simulink model "task3"  (R2023b)
settings: Solver=FixedStepDiscrete  StartTime=0.0  StopTime=120  FixedStep=5e-5  RelTol=1e-3
PreLoadFcn:
  | Simulink.defineIntEnumType('windowCommand', {'Off','Speed1','Speed2','Speed3'},[0,1,2,3])
undefined symbols (not defined in the file or in its folder): designMultirateFIR
libraries: dspmlti4 x1, dspfdesign x1, slpidlib x1
settings Model: Creator=kz1nz0  LastModifiedBy=helme

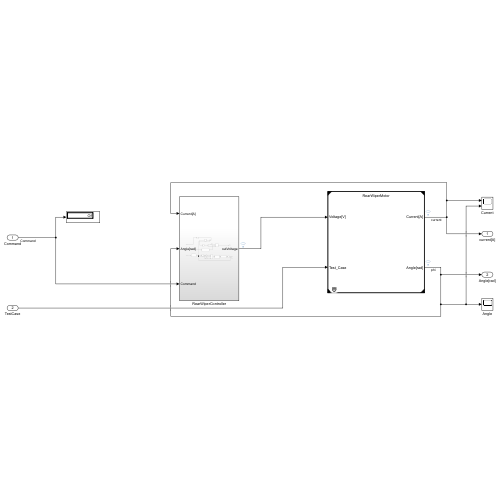
[thumbnail: Simulink's stored preview of the top-level diagram]
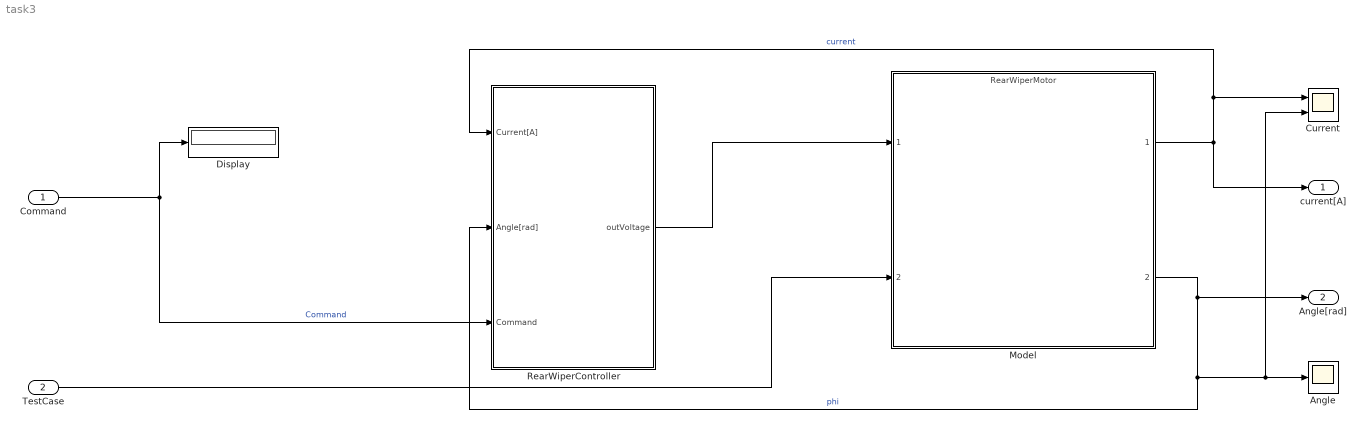
== system task3 ==
  Command : Inport  OutDataTypeStr=Enum: windowCommand
  TestCase : Inport  Port=2  OutDataTypeStr=int8
  Angle : Scope
  Current : Scope  NumInputPorts=2
  Display : Display
  Model : ModelReference  ModelNameDialog=RearWiperMotor.slxp  ModelReferenceVersion=19.15  CopyOfModelProtected=on
  RearWiperController : Subsystem
  current[A] : Outport
  Angle[rad] : Outport  Port=2
  wires:
  TestCase/1 -> Model/2
  Model/1 -> RearWiperController/1(Current[A]), Current/1, current[A]/1  "current"
  Model/2 -> Current/2, Angle/1, RearWiperController/2(Angle[rad]), Angle[rad]/1  "phi"
  RearWiperController/1(outVoltage) -> Model/1
  Command/1 -> Display/1, RearWiperController/3(Command)  "Command"

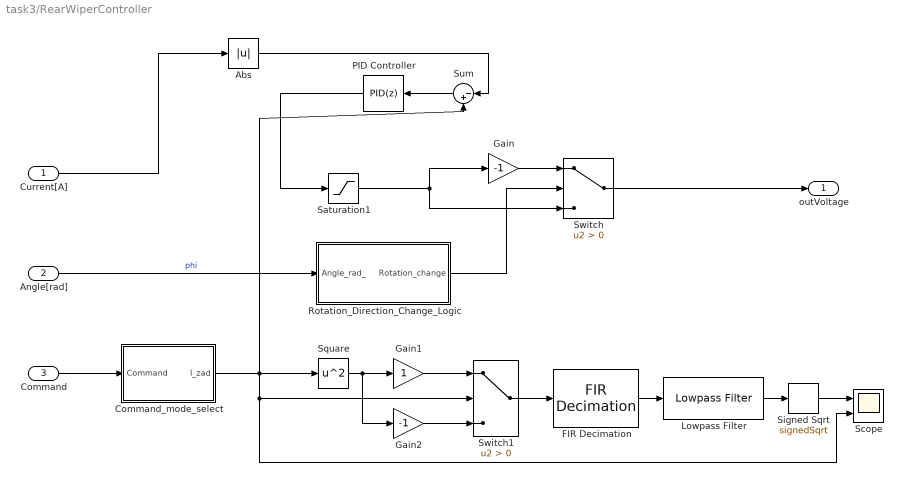
== system task3/RearWiperController ==
  Current[A] : Inport
  Angle[rad] : Inport  Port=2
  Command : Inport  Port=3  OutDataTypeStr=Enum: windowCommand
  Abs : Abs  SaturateOnIntegerOverflow=off
  Command_mode_select : Stateflow chart  TreatAsAtomicUnit=on
  FIR Decimation : dspmlti4/FIR Decimation  FilterSource=Auto  h=designMultirateFIR(1,2)  D=15  filtStruct=Direct form  FilterObject=FDECIM  framing=Enforce single-rate processing  AllowArbitraryInputLength=off  inputOffset=0  outputBufInitCond=0  roundingMode=Floor  overflowMode=off  firstCoeffDataTypeStr=Inherit: Same word length as input  firstCoeffMin=[]  firstCoeffMax=[]  firstCoeffLastDataTypeStr=Inherit: Same word length as input  outputDataTypeStr=Inherit: Same as accumulator  outputMin=[]  outputMax=[]  outputLastDataTypeStr=Inherit: Same as accumulator
  Gain : Gain  Gain=-1
  Gain1 : Gain
  Gain2 : Gain  Gain=-1
  Lowpass Filter : dspfdesign/Lowpass Filter  FilterType=FIR  DesignForMinimumOrder=on  FilterOrder=50  PassbandFrequency=8e3  StopbandFrequency=12e3  PassbandRipple=0.1  StopbandAttenuation=80  SampleRateMode=Specify on dialog  SampleRate=44100  SimulateUsing=Interpreted execution  roundingMode=Floor  coeffsDataTypeStr=fixdt(1,16)
  PID Controller : slpidlib/PID Controller  Controller=PID  Form=Parallel  TimeDomain=Discrete-time  UseExternalTs=off  SampleTime=-1  IntegratorMethod=Forward Euler  FilterMethod=Forward Euler  ControllerParametersSource=internal  P=20  I=0  UseKiTs=off  D=2  N=100  UseFilter=on  TunerSelectOption=Transfer Function Based (PID Tuner App)  InitialConditionSource=internal  InitialConditionForIntegrator=0  InitialConditionForFilter=0  DifferentiatorICPrevScaledInput=0  ExternalReset=none  TrackingMode=off  Kt=1  LimitOutput=off  SatLimitsSource=internal  UpperSaturationLimit=inf  LowerSaturationLimit=-inf  LinearizeAsGain=on  AntiWindupMode=none  Kb=1  LimitIntegrator=off  UpperIntegratorSaturationLimit=inf  LowerIntegratorSaturationLimit=-inf  POutMin=[]  POutMax=[]  IOutMin=[]  IOutMax=[]  DOutMin=[]  DOutMax=[]  NOutMin=[]  NOutMax=[]  SumOutMin=[]  SumOutMax=[]  SaturationOutMin=[]  SaturationOutMax=[]  PParamMin=[]  PParamMax=[]  IParamMin=[]  IParamMax=[]  DParamMin=[]  DParamMax=[]  NParamMin=[]  NParamMax=[]  KbParamMin=[]  KbParamMax=[]  KtParamMin=[]  KtParamMax=[]  KbOutMin=[]  KbOutMax=[]  KtOutMin=[]  KtOutMax=[]  IntegratorOutMin=[]  IntegratorOutMax=[]  FilterOutMin=[]  FilterOutMax=[]  SumI1OutMin=[]  SumI1OutMax=[]  SumI2OutMin=[]  SumI2OutMax=[]  SumI3OutMin=[]  SumI3OutMax=[]  SumI4OutMin=[]  SumI4OutMax=[]  SumDOutMin=[]  SumDOutMax=[]  DifferentiatorOutMin=[]  DifferentiatorOutMax=[]  FilterDiffOutCoefMin=[]  FilterDiffOutCoefMax=[]  ReciprocalOutMin=[]  ReciprocalOutMax=[]  SumDenOutMin=[]  SumDenOutMax=[]  SumNumOutMin=[]  SumNumOutMax=[]  DivideOutMin=[]  DivideOutMax=[]  UdiffTsProdOutMin=[]  UdiffTsProdOutMax=[]  NTsProdOutMin=[]  NTsProdOutMax=[]  UintegralTsProdOutMin=[]  UintegralTsProdOutMax=[]  UngainTsProdOutMin=[]  UngainTsProdOutMax=[]  ClampingZeroOutDataTypeStr=Inherit: Inherit via back propagation  ClampingZeroOutMin=[]  ClampingZeroOutMax=[]  FilterDenConstantOutDataTypeStr=Inherit: Inherit via back propagation  FilterDenConstantOutMin=[]  FilterDenConstantOutMax=[]  PCopyOutDataTypeStr=Inherit: Inherit via back propagation  PCopyOutMin=[]  PCopyOutMax=[]  NCopyOutDataTypeStr=Inherit: Inherit via back propagation  NCopyOutMin=[]  NCopyOutMax=[]  IntegratorContinuousStateAttributes=''  IntegratorStateMustResolveToSignalObject=off  IntegratorRTWStateStorageClass=Auto  FilterContinuousStateAttributes=''  FilterStateMustResolveToSignalObject=off  FilterRTWStateStorageClass=Auto  ParallelPVariant=InternalParameters  IdealPVariant=Disabled  IVariant=InternalParameters  DVariant=InternalParameters  IntegratorVariant=Discrete  SatVariant=Disabled  AWVariant=Passthrough  PCopyVariant=Disabled  TRVariant=Disabled  FdbkBlocksVariant=Forward  IdealPFdbkVariant=Disabled  SatFdbkVariant=Disabled  DerivativeFilterVariant=ForwardEulerFilter  NVariant=InternalParameters  NCopyVariant=Disabled  FilterICVariant=InternalICsFilter  IntegratorICVariant=InternalICs  ExternalResetVariant=Disabled  TRSumVariant=Passthrough  SumFdbkVariant=Disabled  SumVariant=Sum_PID  TsampFilterVariant=InternalTs  TsampNgainVariant=Passthrough  TsampIntegralVariant=Disabled_SignalSpec  ExternalSaturationOutDataTypeStr=Inherit: Same as second input
  Rotation_Direction_Change_Logic : Stateflow chart  TreatAsAtomicUnit=on
  Saturation1 : Saturate  UpperLimit=12  LowerLimit=-12
  Scope : Scope  NumInputPorts=2
  Signed Sqrt : Sqrt  Operator=signedSqrt
  Square : Math  Operator=square
  Sum : Sum  Inputs=|-+
  Switch : Switch  Criteria=u2 > Threshold  SaturateOnIntegerOverflow=off  InputSameDT=off
  Switch1 : Switch  Criteria=u2 > Threshold  SaturateOnIntegerOverflow=off  InputSameDT=off
  outVoltage : Outport
  wires:
  Rotation_Direction_Change_Logic/1(Rotation_change) -> Switch/2
  Gain/1 -> Switch/1
  Command/1 -> Command_mode_select/1(Command)
  Angle[rad]/1 -> Rotation_Direction_Change_Logic/1(Angle_rad_)  "phi"
  Saturation1/1 -> Switch/3, Gain/1
  Sum/1 -> PID Controller/1
  PID Controller/1 -> Saturation1/1
  Switch/1 -> outVoltage/1
  Abs/1 -> Sum/1
  Current[A]/1 -> Abs/1
  Command_mode_select/1(I_zad) -> Scope/2, Switch1/2, Square/1, Sum/2
  Square/1 -> Gain2/1, Gain1/1
  Gain2/1 -> Switch1/3
  Gain1/1 -> Switch1/1
  Switch1/1 -> FIR Decimation/1
  FIR Decimation/1 -> Lowpass Filter/1
  Lowpass Filter/1 -> Signed Sqrt/1
  Signed Sqrt/1 -> Scope/1

== stateflow chart task3/RearWiperController/Command_mode_select ==
  state Off
    entry:
    I_zad = 0;
  state first_speed
    entry:
    I_zad = 9;
  state third_speed
    entry:
    I_zad = 3;
  state second_speed
    entry:
    I_zad = 6;
  (default) -> Off
  Off -> third_speed [order 3] : [Command == 3]
  Off -> first_speed [order 1] : [Command == 1]
  first_speed -> Off [order 1] : [Command == 0]
  third_speed -> Off [order 1] : [Command == 0]
  second_speed -> Off [order 2] : [Command == 0]
  Off -> second_speed [order 2] : [Command == 2]
  second_speed -> first_speed [order 1] : [Command == 1]
  third_speed -> first_speed [order 2] : [Command == 1]
  first_speed -> third_speed [order 3] : [Command == 3]
  first_speed -> second_speed [order 2] : [Command == 2]
  second_speed -> third_speed [order 3] : [Command == 3]
  third_speed -> second_speed [order 3] : [Command == 2]
  data: Command input; I_zad output

== stateflow chart task3/RearWiperController/Rotation_Direction_Change_Logic ==
  state KIERUNEK_CW
    entry:
    Rotation_change = 0;
  state KIERUNEK_CCW
    entry:
    Rotation_change = 1;
  (default) -> KIERUNEK_CW
  KIERUNEK_CCW -> KIERUNEK_CW : [Angle_rad_<=1.05]
  KIERUNEK_CW -> KIERUNEK_CCW : [Angle_rad_>=1.95]
  data: Angle_rad_ input; Rotation_change output =0; kat local
